simulink model "dc_motor"  (R2015a)
settings: Solver=ode3  StartTime=0.0  StopTime=10.0  FixedStep=0.001  RelTol=1e-3
values from neighbouring files (symbols this model uses):
  b = 50    [cruise_control_ss.m]
undefined symbols (not defined in the file or in its folder): J, K, L, R
settings Model: Creator=Xiaotian  LastModifiedBy=Xiaotian

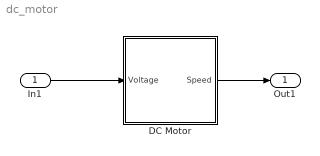
== system dc_motor ==
  In1 : Inport
  DC Motor : Subsystem
  Out1 : Outport
  wires:
  DC Motor/1(Speed) -> Out1/1
  In1/1 -> DC Motor/1(Voltage)

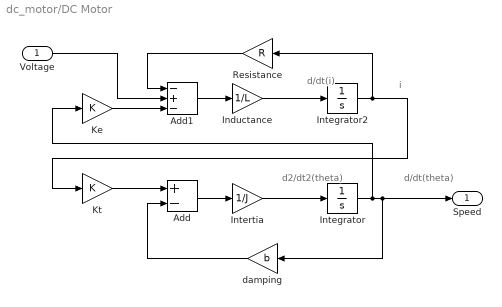
== system dc_motor/DC Motor ==
  note: i
  note: d/dt(theta)
  note: d2/dt2(theta)
  note: d/dt(i)
  Voltage : Inport
  Add : Sum  Inputs=+-
  Add1 : Sum  Inputs=-+-
  Inductance : Gain  Gain=1/L
  Integrator : Integrator
  Integrator2 : Integrator
  Intertia : Gain  Gain=1/J
  Ke : Gain  Gain=K
  Kt : Gain  Gain=K
  Resistance : Gain  Gain=R
  damping : Gain  Gain=b
  Speed : Outport
  wires:
  Inductance/1 -> Integrator2/1
  Integrator/1 -> Speed/1, damping/1, Ke/1
  Intertia/1 -> Integrator/1
  Integrator2/1 -> Kt/1, Resistance/1
  Add/1 -> Intertia/1
  Add1/1 -> Inductance/1
  Kt/1 -> Add/1
  damping/1 -> Add/2
  Ke/1 -> Add1/3
  Resistance/1 -> Add1/1
  Voltage/1 -> Add1/2
